simulink model "Sim_Force2Motion_Model"  (Simulink 7.4)
settings: Solver=ode45  StartTime=0.0  StopTime=tsimend  MaxStep=0.01  RelTol=1e-3
undefined symbols (not defined in the file): A_inf, A_IRF, B_IRF, C_IRF, D_IRF, G, M
settings Model: Creator=Taha  LastModifiedBy=Taha

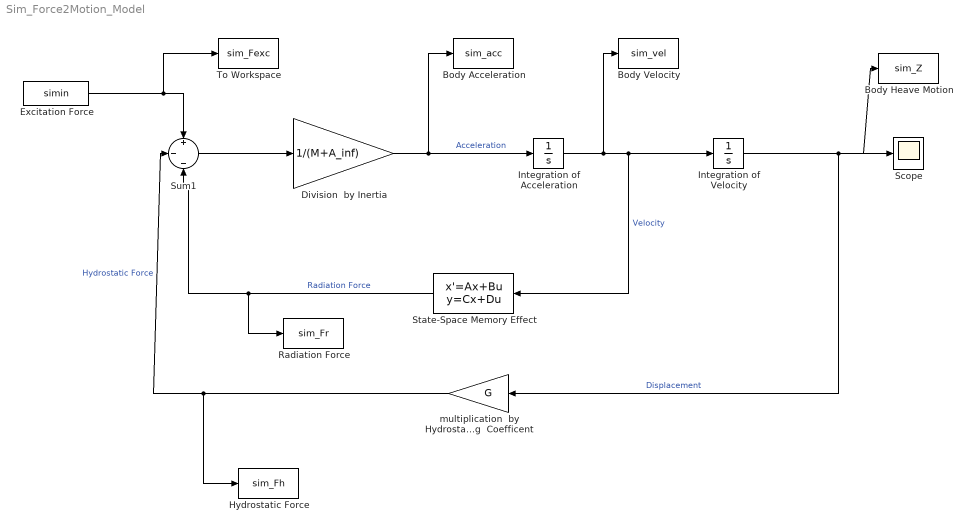
== system Sim_Force2Motion_Model ==
  Body Heave Motion : ToWorkspace  VariableName=sim_Z  SampleTime=-1  SaveFormat=Structure With Time
  Body Acceleration : ToWorkspace  VariableName=sim_acc  SampleTime=-1  SaveFormat=Structure With Time
  Body Velocity : ToWorkspace  VariableName=sim_vel  SampleTime=-1  SaveFormat=Structure With Time
  Division  by Inertia : Gain  Gain=1/(M+A_inf)  ParameterDataType=fixdt(1, 16)  ParameterScaling=2^0  OutDataType=fixdt(1, 16)  OutScaling=2^0
  Excitation Force : FromWorkspace  VariableName=simin  SampleTime=0
  Hydrostatic Force : ToWorkspace  VariableName=sim_Fh  SampleTime=-1  SaveFormat=Structure With Time
  Integration of Acceleration : Integrator
  Integration of Velocity : Integrator
  Radiation Force : ToWorkspace  VariableName=sim_Fr  SampleTime=-1  SaveFormat=Structure With Time
  Scope : Scope
  State-Space Memory Effect : StateSpace  A=A_IRF  B=B_IRF  C=C_IRF  D=D_IRF
  Sum1 : Sum  Inputs=+|-|-  OutDataType=fixdt(1, 16)  OutScaling=2^0
  To Workspace : ToWorkspace  VariableName=sim_Fexc  SampleTime=-1  SaveFormat=Structure With Time
  multiplication  by Hydrostatic Restoring  Coefficent : Gain  Gain=G  ParameterDataType=fixdt(1, 16)  ParameterScaling=2^0  OutDataType=fixdt(1, 16)  OutScaling=2^0
  wires:
  Integration of Acceleration/1 -> Integration of Velocity/1, State-Space Memory Effect/1, Body Velocity/1  "Velocity"
  Integration of Velocity/1 -> multiplication  by Hydrostatic Restoring  Coefficent/1, Scope/1, Body Heave Motion/1  "Displacement"
  Division  by Inertia/1 -> Integration of Acceleration/1, Body Acceleration/1  "Acceleration"
  State-Space Memory Effect/1 -> Radiation Force/1, Sum1/3  "Radiation Force"
  Sum1/1 -> Division  by Inertia/1
  multiplication  by Hydrostatic Restoring  Coefficent/1 -> Hydrostatic Force/1, Sum1/2  "Hydrostatic Force"
  Excitation Force/1 -> Sum1/1, To Workspace/1
